simulink model "Sim_XZ"  (R2016a)
settings: Solver=VariableStepAuto  StartTime=0.0  StopTime=10.0  RelTol=1e-3
values from neighbouring files (symbols this model uses):
  k_reg = 0.672    [Systemdesign_XY.m]
  k_s = double(subs(k_s,T_z,1))    [Systemdesign_XY.m]
  T_n1 = 0.1    [Systemdesign_XY.m]
  T_n2 = 1/12    (= 0.0833333333333)    [Systemdesign_XY.m]
  T_v = 0.2    [Systemdesign_XY.m]
settings Model: Creator=Florian  LastModifiedBy=Florian

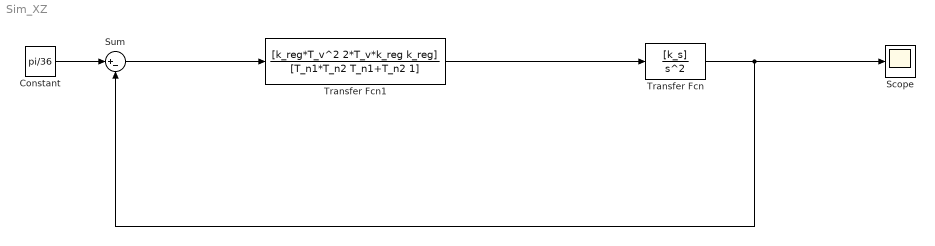
== system Sim_XZ ==
  Constant : Constant  Value=pi/36
  Scope : Scope
  Sum : Sum  Inputs=|+-
  Transfer Fcn : TransferFcn  Numerator=[k_s]  Denominator=[1 0 0]
  Transfer Fcn1 : TransferFcn  Numerator=[k_reg*T_v^2 2*T_v*k_reg k_reg]  Denominator=[T_n1*T_n2 T_n1+T_n2 1]
  wires:
  Transfer Fcn/1 -> Scope/1, Sum/2
  Sum/1 -> Transfer Fcn1/1
  Constant/1 -> Sum/1
  Transfer Fcn1/1 -> Transfer Fcn/1
